simulink model "data"  (R2024b)
settings: Solver=ode4  StartTime=0.0  StopTime=simulation_time  FixedStep=sample_time  RelTol=1e-3
values from neighbouring files (symbols this model uses):
  init_dq = initial(i).init_dq    [err_percentage_calculator.m]
  init_q = initial(i).init_q    [err_percentage_calculator.m]
settings Model: Creator=zhes  LastModifiedBy=zhes

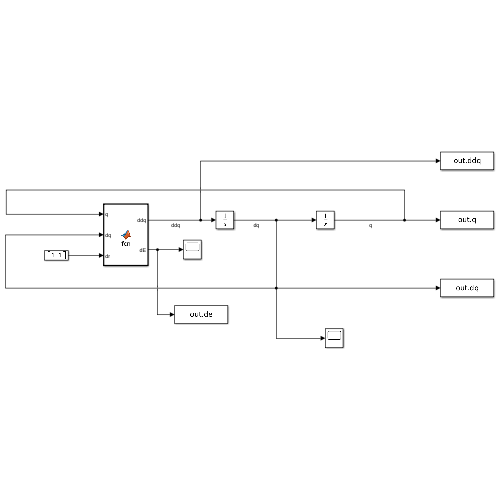
[thumbnail: Simulink's stored preview of the top-level diagram]
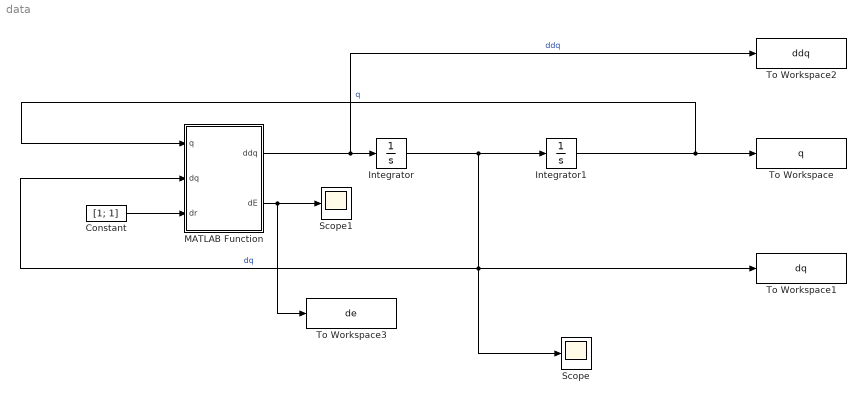
== system data ==
  Constant : Constant  Value=[1; 1]
  Integrator : Integrator  InitialCondition=init_dq
  Integrator1 : Integrator  InitialCondition=init_q
  MATLAB Function : MATLAB Function  TreatAsAtomicUnit=on
  Scope : Scope
  Scope1 : Scope
  To Workspace : ToWorkspace  VariableName=q  SaveFormat=Structure With Time  SampleTime=-1
  To Workspace1 : ToWorkspace  VariableName=dq  SaveFormat=Structure With Time  SampleTime=-1
  To Workspace2 : ToWorkspace  VariableName=ddq  SaveFormat=Structure With Time  SampleTime=-1
  To Workspace3 : ToWorkspace  VariableName=de  SaveFormat=Structure With Time  SampleTime=-1
  wires:
  Integrator/1 -> MATLAB Function/2(dq), To Workspace1/1, Scope/1, Integrator1/1  "dq"
  Integrator1/1 -> To Workspace/1, MATLAB Function/1(q)  "q"
  MATLAB Function/1(ddq) -> To Workspace2/1, Integrator/1  "ddq"
  Constant/1 -> MATLAB Function/3(dr)
  MATLAB Function/2(dE) -> To Workspace3/1, Scope1/1

== matlab function data/MATLAB Function ==
  data: q input; ddq output; dq input; dr input; dE output
function [ddq, dE]= fcn(q, dq, dr)

q1 = q(1);
q2 = q(2);
dq1 = dq(1);
dq2 = dq(2);

dr1 = dr(1);
dr2 = dr(2);

kD = diag([10,10]);

Gq = [ cos(q1) + cos(q1 + q2);
       cos(q1 + q2)];

de1 = dr1 - dq1;
de2 = dr2 - dq2;

dE = [de1; de2];

ddq = -dq - Gq + kD * dE;
